simulink model "DynamicWeightCalculationModel"  (R2014a)
settings: Solver=ode45  StartTime=0.0  StopTime=100  RelTol=1e-3
settings Model: CovSFcnEnable=on  Creator=shawn  LastModifiedBy=scorpii
settings DebuggingCC: MergeDetectMultiDrivingBlocksExec=error  SolverPrmCheckMsg=none  FrameProcessingCompatibilityMsg=error

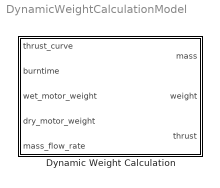
== system DynamicWeightCalculationModel ==
  Dynamic Weight Calculation : Subsystem

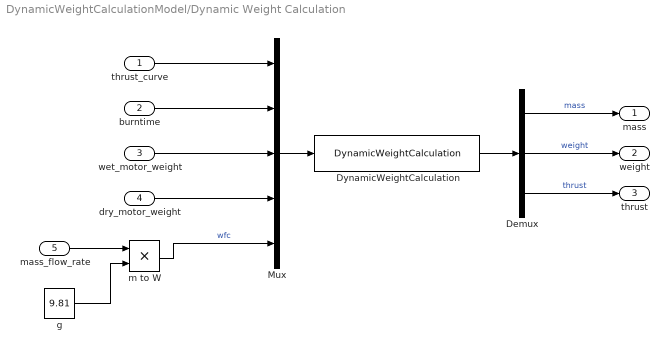
== system DynamicWeightCalculationModel/Dynamic Weight Calculation ==
  thrust_curve : Inport
  burntime : Inport  Port=2
  wet_motor_weight : Inport  Port=3
  dry_motor_weight : Inport  Port=4
  mass_flow_rate : Inport  Port=5
  Demux : Demux  Outputs=[1 1 1]
  DynamicWeightCalculation : MATLABFcn  MATLABFcn=DynamicWeightCalculation
      mask Display: disp('DynamicWeightCalculation')
  Mux : Mux  Inputs=5
  g : Constant  Value=9.81
  m to W : Product
  mass : Outport
  weight : Outport  Port=2
  thrust : Outport  Port=3
  wires:
  burntime/1 -> Mux/2
  Demux/1 -> mass/1  "mass"
  Demux/2 -> weight/1  "weight"
  Mux/1 -> DynamicWeightCalculation/1
  DynamicWeightCalculation/1 -> Demux/1
  Demux/3 -> thrust/1  "thrust"
  mass_flow_rate/1 -> m to W/1
  g/1 -> m to W/2
  m to W/1 -> Mux/5  "wfc"
  wet_motor_weight/1 -> Mux/3
  thrust_curve/1 -> Mux/1
  dry_motor_weight/1 -> Mux/4
